simulink model "week3_prob2"  (R2020b)
settings: Solver=VariableStepAuto  StartTime=0.0  StopTime=10.0  RelTol=1e-3
settings Model: Creator=varunraj  LastModifiedBy=varunraj

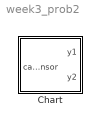
== system week3_prob2 ==
  Chart : Stateflow chart  TreatAsAtomicUnit=on

== stateflow chart week3_prob2/Chart ==
  state Stop
    en:y1=red;
    y2=green;
  state Stop_Traffic
    en:
    y1=red;
    y2=green;
  state Stop_Go
    en:
    y1=red;
    y2=yellow;
  state Go_Stop
    en:
    y1=yellow;
    y2=red;
  state Go
    en:
    y1=green;
    y2=red;
  (default) -> Stop
  Stop -> Stop_Traffic : after(10,sec)
  Go_Stop -> Stop : after(5,sec)
  Stop_Traffic -> Stop_Go : [car_sensor]
  Stop_Go -> Go : after(5,sec)
  Go -> Go_Stop : after(10,sec)
  data: green constant double =3; yellow constant double =2; red constant double =1; y1 output; car_sensor input; y2 output
